simulink model "stereo_ibvs_core_before_04_kinematics_20260723_212009"  (R2025b)
settings: Solver=FixedStepDiscrete  StartTime=0.0  StopTime=inf  FixedStep=cfg.Ts  RelTol=1e-3
InitFcn:
  | cfgValid__=evalin('base','exist(''cfg'',''var'')==1 && isstruct(cfg) && all(isfield(cfg,{''Ts'',''robot'',''qInitial'',''zoomInitialSteps'',''cameraIntrinsicsStage1'',''rhoD'',''stereoBaseline'',''centerDesired'',''Kc'',''lambdaC'',''qMin'',''qMax'',''qLimitSoftMargin'',''qDotAlgorithmMax'',''stage1CalibrationReady''}))');if ~cfgValid__,modelFile__=get_param(bdroot,'FileName');modelDir__=fileparts(modelFile__);config1__=fullfile(modelDir__,'stereo_ibvs_config.m');config2__=fullfile(fileparts(modelDir__),'config','stereo_ibvs_config.m');if isfile(config1__),run(config1__);elseif isfile(config2__),run(config2__);else,error('StereoIBVS:ConfigNotFound','找不到stereo_ibvs_config.m。');end;end;clear cfgValid__ modelFile__ modelDir__ config1__ config2__
undefined symbols (not defined in the file): cfg
(part 2 of 2)

== matlab function stereo_ibvs_core_before_04_kinematics_20260723_212009/08_Zoom_Controller/08C Zoom Priority Supervisor ==
  data: scaleError input; depthErrorDelayed input; focalLengthMeasuredMm input; focalAtWorkingLowerLimit input; focalAtWorkingUpperLimit input; depthTaskWeight output; focalHeadroomMm input; focalFeasible input; validLeft input; validStereoQualified input; ekfPredictionValid input; resetSafe input; focalCommandOutwardAtWorkingLimit input; focalRateUsageGuaranteedCmd input; focalRateUsageHardCmd input; rightReacquireActive input; schedulerMode output; zoomPriorityActive output; zoomPriorityTimer output; scaleSettledTimer output; armRecoveryReason output; newDisturbanceDetected output
function [ ...
    depthTaskWeight, ...
    schedulerMode, ...
    zoomPriorityActive, ...
    zoomPriorityTimer, ...
    scaleSettledTimer, ...
    armRecoveryReason, ...
    newDisturbanceDetected] = fcn( ...
    scaleError, ...
    depthErrorDelayed, ...
    focalLengthMeasuredMm, ...
    focalAtWorkingLowerLimit, ...
    focalAtWorkingUpperLimit, ...
    focalHeadroomMm, ...
    focalFeasible, ...
    validLeft, ...
    validStereoQualified, ...
    ekfPredictionValid, ...
    resetSafe, ...
    focalCommandOutwardAtWorkingLimit, ...
    focalRateUsageGuaranteedCmd, ...
    focalRateUsageHardCmd, ...
    rightReacquireActive)
%#codegen
% V2 Zoom优先级状态机。
%
% schedulerMode:
% 0 INITIALIZE
% 1 ZOOM_FIRST
% 2 ARM_RECOVERY
% 3 FULL_TRACK
% 4 SAFE_HOLD
% 5 RIGHT_REACQUIRE

persistent mode
persistent zoomTimer
persistent settledTimer
persistent rampTimer
persistent reason
persistent disturbanceTimer
persistent validLast
persistent rateTimer

if isempty(mode)
    mode = 0;
    zoomTimer = 0;
    settledTimer = 0;
    rampTimer = 0;
    reason = 0;
    disturbanceTimer = 0;
    validLast = 0;
    rateTimer = 0;
end

if resetSafe > 0.5
    mode = 0;
    zoomTimer = 0;
    settledTimer = 0;
    rampTimer = 0;
    reason = 0;
    disturbanceTimer = 0;
    validLast = 0;
    rateTimer = 0;
end

depthTaskWeight = 0;
newDisturbanceDetected = 0;

centerValid = validLeft > 0.5;

depthReady = ...
    validStereoQualified > 0.5 && ...
    ekfPredictionValid > 0.5 && ...
    rightReacquireActive <= 0.5;

maximumScaleError = max(abs(scaleError));

if ~centerValid

    mode = 4;
    depthTaskWeight = 0;
    validLast = 0;

elseif ~depthReady

    mode = 5;
    depthTaskWeight = 0;
    validLast = 0;
    rampTimer = 0;

elseif cfg_zoomPriorityEnable <= 0.5

    mode = 3;
    depthTaskWeight = 1;

    zoomTimer = 0;
    settledTimer = 0;
    rampTimer = cfg_armDepthRampTime;

    reason = 0;
    disturbanceTimer = 0;
    validLast = 1;

else

    if validLast < 0.5 && ...
            (mode == 4 || mode == 5)

        mode = 1;

        zoomTimer = 0;
        settledTimer = 0;
        rampTimer = 0;

        reason = 0;
        disturbanceTimer = 0;
    end

    if mode == 0

        if maximumScaleError > ...
                cfg_scaleErrorEnterThreshold

            mode = 1;
            depthTaskWeight = 0;
        else
            mode = 3;
            depthTaskWeight = 1;
        end

    elseif mode == 1

        depthTaskWeight = 0;
        zoomTimer = zoomTimer + cfg_Ts;

        if maximumScaleError <= ...
                cfg_scaleErrorExitThreshold

            settledTimer = settledTimer + cfg_Ts;
        else
            settledTimer = 0;
        end

        if any(focalRateUsageGuaranteedCmd >= 1)
            rateTimer = rateTimer + cfg_Ts;
        else
            rateTimer = 0;
        end

        if any(focalRateUsageHardCmd >= 1)

            mode = 2;
            reason = 6;
            rampTimer = 0;

        elseif rateTimer >= ...
                cfg_disturbanceConfirmTime && ...
                maximumScaleError > ...
                cfg_scaleErrorExitThreshold

            mode = 2;
            reason = 5;
            rampTimer = 0;

        elseif settledTimer >= ...
                cfg_scaleSettledHoldTime

            mode = 2;
            reason = 1;
            rampTimer = 0;

        elseif any( ...
                focalCommandOutwardAtWorkingLimit > 0.5)

            mode = 2;
            reason = 7;
            rampTimer = 0;

        elseif zoomTimer >= ...
                cfg_disturbanceConfirmTime && ...
                any(focalFeasible < 0.5)

            mode = 2;
            reason = 3;
            rampTimer = 0;

        elseif zoomTimer >= cfg_zoomOnlyMaxTime

            mode = 2;
            reason = 4;
            rampTimer = 0;
        end

    elseif mode == 2

        rampTimer = min( ...
            rampTimer + cfg_Ts, ...
            cfg_armDepthRampTime);

        rampFraction = min(max( ...
            rampTimer / max( ...
                cfg_armDepthRampTime, ...
                cfg_Ts), ...
            0), 1);

        depthTaskWeight = ...
            rampFraction * rampFraction * ...
            (3 - 2*rampFraction);

        if depthTaskWeight >= 1 - 1e-6
            mode = 3;
            depthTaskWeight = 1;
            disturbanceTimer = 0;
        end

    elseif mode == 3

        depthTaskWeight = 1;

        if maximumScaleError >= ...
                cfg_scaleErrorEnterThreshold

            depthTaskWeight = 0;
            disturbanceTimer = ...
                disturbanceTimer + cfg_Ts;
        else
            disturbanceTimer = 0;
        end

        if disturbanceTimer >= ...
                cfg_disturbanceConfirmTime

            mode = 1;
            depthTaskWeight = 0;

            zoomTimer = 0;
            settledTimer = 0;
            rampTimer = 0;

            reason = 0;
            disturbanceTimer = 0;

            newDisturbanceDetected = 1;
        end

    else

        mode = 1;
        depthTaskWeight = 0;

        zoomTimer = 0;
        settledTimer = 0;
        rampTimer = 0;

        reason = 0;
    end

    validLast = 1;
end

schedulerMode = mode;
zoomPriorityActive = double(mode == 1);

zoomPriorityTimer = zoomTimer;
scaleSettledTimer = settledTimer;
armRecoveryReason = reason;

%% 数值保护
if any(~isfinite([
        depthTaskWeight
        schedulerMode
        zoomPriorityTimer
        scaleSettledTimer
        depthErrorDelayed
        focalLengthMeasuredMm
        focalHeadroomMm
        focalAtWorkingLowerLimit
        focalAtWorkingUpperLimit]))

    depthTaskWeight = 0;
    schedulerMode = 4;
    zoomPriorityActive = 0;
    newDisturbanceDetected = 0;
end
end

== matlab function stereo_ibvs_core_before_04_kinematics_20260723_212009/04_FR3_Camera_Kinematics/Express Jacobian in Left Camera ==
  data: q input; pWCL output; cfg_T_W_B input; cfg_fr3OriginXYZ input; cfg_fr3OriginRPY input; cfg_fr3Axis input; cfg_fr3Joint8OriginXYZ input; cfg_fr3Joint8OriginRPY input; cfg_T_link8_CL input; cfg_T_CL_CR input; cfg_numericalEpsilon input; RWCL output; pWCR output; RWCR output; JL output; JR output; kinematicsValid output
function [ ...
    pWCL, ...
    RWCL, ...
    pWCR, ...
    RWCR, ...
    JL, ...
    JR, ...
    kinematicsValid] = fcn(q, cfg_T_W_B, cfg_fr3OriginXYZ, cfg_fr3OriginRPY, cfg_fr3Axis, cfg_fr3Joint8OriginXYZ, cfg_fr3Joint8OriginRPY, cfg_T_link8_CL, cfg_T_CL_CR, cfg_numericalEpsilon)
%#codegen
% V2 FR3双目相机运动学。
%
% 输入：
% q：FR3七关节角，7×1，单位rad。
%
% 输出：
% pWCL、RWCL：左相机在世界坐标系中的位置和姿态。
% pWCR、RWCR：右相机在世界坐标系中的位置和姿态。
% JL、JR：左右相机坐标系表达的相机Jacobian，
%          排列顺序为[线速度; 角速度]。
% kinematicsValid：运动学结果是否有效。

%% 固定尺寸输出初始化
pWCL = zeros(3,1);
RWCL = eye(3);

pWCR = zeros(3,1);
RWCR = eye(3);

JL = zeros(6,7);
JR = zeros(6,7);

kinematicsValid = false;

%% 输入检查
if any(~isfinite(q))
    return;
end

%% FR3正运动学
T = cfg_T_W_B;

jointOriginsW = zeros(3,7);
jointAxesW = zeros(3,7);

for jointIndex = 1:7

    % 当前关节固定原点变换
    T = T * makeTransform( ...
        cfg_fr3OriginXYZ(:,jointIndex), ...
        cfg_fr3OriginRPY(:,jointIndex));

    jointOriginsW(:,jointIndex) = T(1:3,4);

    axisLocal = cfg_fr3Axis(:,jointIndex);
    axisNorm = norm(axisLocal);

    if ~isfinite(axisNorm) || ...
            axisNorm <= cfg_numericalEpsilon
        return;
    end

    jointAxesW(:,jointIndex) = ...
        T(1:3,1:3) * axisLocal;

    % 当前关节转动
    T = T * axisRotation(axisLocal,q(jointIndex));
end

%% link8固定变换
T_W_link8 = T * makeTransform( ...
    cfg_fr3Joint8OriginXYZ, ...
    cfg_fr3Joint8OriginRPY);

%% 左右相机位姿
T_W_CL = T_W_link8 * cfg_T_link8_CL;
T_W_CR = T_W_CL * cfg_T_CL_CR;

pWCL = T_W_CL(1:3,4);
RWCL = T_W_CL(1:3,1:3);

pWCR = T_W_CR(1:3,4);
RWCR = T_W_CR(1:3,1:3);

%% 左相机光心世界坐标Jacobian
JWLeft = zeros(6,7);

for jointIndex = 1:7

    JWLeft(1:3,jointIndex) = cross( ...
        jointAxesW(:,jointIndex), ...
        pWCL-jointOriginsW(:,jointIndex));

    JWLeft(4:6,jointIndex) = ...
        jointAxesW(:,jointIndex);
end

%% 转换到左相机坐标系
R_CL_W = RWCL';

JL = [
    R_CL_W, zeros(3,3)
    zeros(3,3), R_CL_W
    ] * JWLeft;

%% 从左相机Jacobian转换为右相机Jacobian
R_CL_CR = cfg_T_CL_CR(1:3,1:3);
p_CL_CR = cfg_T_CL_CR(1:3,4);

JR = [
    R_CL_CR', -R_CL_CR' * skew3(p_CL_CR)
    zeros(3,3), R_CL_CR'
    ] * JL;

%% 有限值和旋转矩阵检查
if any(~isfinite(pWCL)) || ...
        any(~isfinite(RWCL(:))) || ...
        any(~isfinite(pWCR)) || ...
        any(~isfinite(RWCR(:))) || ...
        any(~isfinite(JL(:))) || ...
        any(~isfinite(JR(:)))

    pWCL = zeros(3,1);
    RWCL = eye(3);
    pWCR = zeros(3,1);
    RWCR = eye(3);
    JL = zeros(6,7);
    JR = zeros(6,7);
    return;
end

rotationTolerance = max( ...
    1e-6, ...
    100*cfg_numericalEpsilon);

if norm(RWCL'*RWCL-eye(3),'fro') > rotationTolerance || ...
        norm(RWCR'*RWCR-eye(3),'fro') > rotationTolerance || ...
        abs(det(RWCL)-1) > rotationTolerance || ...
        abs(det(RWCR)-1) > rotationTolerance
    return;
end

kinematicsValid = true;

end


function T = makeTransform(xyz,rpy)

T = eye(4);

T(1:3,1:3) = ...
    rotz3(rpy(3)) * ...
    roty3(rpy(2)) * ...
    rotx3(rpy(1));

T(1:3,4) = xyz;

end


function T = axisRotation(axis,q)

axisNorm = norm(axis);
unitAxis = axis / axisNorm;

K = skew3(unitAxis);

R = eye(3) + ...
    sin(q)*K + ...
    (1-cos(q))*(K*K);

T = eye(4);
T(1:3,1:3) = R;

end


function R = rotx3(angle)

c = cos(angle);
s = sin(angle);

R = [
    1, 0, 0
    0, c, -s
    0, s, c
    ];

end


function R = roty3(angle)

c = cos(angle);
s = sin(angle);

R = [
    c, 0, s
    0, 1, 0
    -s, 0, c
    ];

end


function R = rotz3(angle)

c = cos(angle);
s = sin(angle);

R = [
    c, -s, 0
    s, c, 0
    0, 0, 1
    ];

end


function S = skew3(vector)

S = [
    0, -vector(3), vector(2)
    vector(3), 0, -vector(1)
    -vector(2), vector(1), 0
    ];

end

== matlab function stereo_ibvs_core_before_04_kinematics_20260723_212009/03_Feature_Processing/Normalize and Validate Features ==
  data: normalizedFeatureMeasured output size=[4 1]; pixelMeasurement input size=[4 1]; cLMeasured output size=[2 1]; scaleMeasuredRaw input size=[2 1]; cRMeasured output size=[2 1]; scaleMeasured output size=[2 1]; zMeasured output size=[3 1]; fxMeasuredPx input size=[2 1]; fyMeasuredPx input size=[2 1]; validLeft input size=[1 1]; validRight input size=[1 1]; visionMeasurementNew input size=[1 1]; resetSafe input size=[1 1]; xLeftMeasured output size=[1 1]; yLeftMeasured output size=[1 1]; xRightMeasured output size=[1 1]; disparityNormalized output size=[1 1]; rhoMeasured output size=[1 1]; validDisparity output size=[1 1]; stereoMeasurementEnable output size=[1 1]; validStereoQualified output size=[1 1]; rightReacquireActive output size=[1 1]; rightReacquireCount output size=[1 1]; uRightMeasured output size=[1 1]
function [ ...
    normalizedFeatureMeasured, ...
    cLMeasured, ...
    cRMeasured, ...
    scaleMeasured, ...
    zMeasured, ...
    xLeftMeasured, ...
    yLeftMeasured, ...
    xRightMeasured, ...
    disparityNormalized, ...
    rhoMeasured, ...
    validDisparity, ...
    stereoMeasurementEnable, ...
    validStereoQualified, ...
    rightReacquireActive, ...
    rightReacquireCount, ...
    uRightMeasured] = fcn( ...
    pixelMeasurement, ...
    scaleMeasuredRaw, ...
    fxMeasuredPx, ...
    fyMeasuredPx, ...
    validLeft, ...
    validRight, ...
    visionMeasurementNew, ...
    resetSafe)
%#codegen
% V2实机视觉测量提取与双目有效性管理。
%
% pixelMeasurement:
% [uL; vL; uR; vR]
%
% scaleMeasuredRaw:
% [scaleL; scaleR]
%
% fxMeasuredPx:
% [fxL; fxR]
%
% fyMeasuredPx:
% [fyL; fyR]
%
% zMeasured:
% [xLeftMeasured; yLeftMeasured; rhoMeasured]

%% 固定尺寸输出
normalizedFeatureMeasured = zeros(4,1);

cLMeasured = zeros(2,1);
cRMeasured = zeros(2,1);
scaleMeasured = zeros(2,1);

zMeasured = zeros(3,1);

xLeftMeasured = 0;
yLeftMeasured = 0;
xRightMeasured = 0;

disparityNormalized = 0;
rhoMeasured = 0;

validDisparity = 0;
stereoMeasurementEnable = 0;
validStereoQualified = 0;

rightReacquireActive = 0;
rightReacquireCount = 0;

uRightMeasured = 0;

%% 右相机重捕获状态
persistent consecutiveValid reacquire

if isempty(consecutiveValid)
    consecutiveValid = 0;
    reacquire = 1;
end

%% 输入整理
pixels = reshape(pixelMeasurement,4,1);
scales = reshape(scaleMeasuredRaw,2,1);
fx = reshape(fxMeasuredPx,2,1);
fy = reshape(fyMeasuredPx,2,1);

inputFinite = ...
    all(isfinite(pixels)) && ...
    all(isfinite(scales)) && ...
    all(isfinite(fx)) && ...
    all(isfinite(fy));

if inputFinite
    uL = pixels(1);
    vL = pixels(2);
    uR = pixels(3);
    vR = pixels(4);

    uRightMeasured = uR;

    leftIntrinsicsValid = ...
        fx(1) > cfg_numericalEpsilon && ...
        fy(1) > cfg_numericalEpsilon;

    rightIntrinsicsValid = ...
        fx(2) > cfg_numericalEpsilon && ...
        fy(2) > cfg_numericalEpsilon;

    leftFeatureValid = ...
        validLeft > 0.5 && ...
        leftIntrinsicsValid;

    rightFeatureValid = ...
        validRight > 0.5 && ...
        rightIntrinsicsValid;

    %% 像素坐标归一化
    if leftIntrinsicsValid
        cLMeasured = [
            (uL - cfg_cxL) / fx(1)
            (vL - cfg_cyL) / fy(1)
        ];
    end

    if rightIntrinsicsValid
        cRMeasured = [
            (uR - cfg_cxR) / fx(2)
            (vR - cfg_cyR) / fy(2)
        ];
    end

    if leftFeatureValid && scales(1) > 0
        scaleMeasured(1) = scales(1);
    end

    if rightFeatureValid && scales(2) > 0
        scaleMeasured(2) = scales(2);
    end

    normalizedFeatureMeasured = [
        cLMeasured
        cRMeasured
    ];

    xLeftMeasured = cLMeasured(1);
    yLeftMeasured = cLMeasured(2);
    xRightMeasured = cRMeasured(1);

    %% 双目视差与逆深度测量
    disparityNormalized = ...
        xLeftMeasured - xRightMeasured;

    candidateRho = 0;

    if cfg_baseline > cfg_numericalEpsilon
        candidateRho = ...
            disparityNormalized / cfg_baseline;
    end

    validDisparity = double( ...
        leftFeatureValid && ...
        rightFeatureValid && ...
        isfinite(candidateRho) && ...
        disparityNormalized > cfg_disparityMin && ...
        candidateRho >= cfg_rhoMin && ...
        candidateRho <= cfg_rhoMax);

    if validDisparity > 0.5
        rhoMeasured = candidateRho;
    end

    zMeasured = [
        xLeftMeasured
        yLeftMeasured
        rhoMeasured
    ];
end

%% 最终有限值保护
if any(~isfinite(normalizedFeatureMeasured))
    normalizedFeatureMeasured = zeros(4,1);
    cLMeasured = zeros(2,1);
    cRMeasured = zeros(2,1);

    zMeasured = zeros(3,1);

    xLeftMeasured = 0;
    yLeftMeasured = 0;
    xRightMeasured = 0;

    disparityNormalized = 0;
    rhoMeasured = 0;
    validDisparity = 0;
end

%% 双目资格与右相机重捕获管理
rawStereoValid = ...
    inputFinite && ...
    validLeft > 0.5 && ...
    validRight > 0.5 && ...
    validDisparity > 0.5;

if resetSafe > 0.5
    consecutiveValid = 0;
    reacquire = 1;

elseif visionMeasurementNew > 0.5
    if rawStereoValid
        consecutiveValid = min( ...
            consecutiveValid + 1, ...
            cfg_rightReacquireValidSamples);
    else
        consecutiveValid = 0;
    end

    if ~rawStereoValid
        reacquire = 1;
    elseif consecutiveValid >= ...
            cfg_rightReacquireValidSamples
        reacquire = 0;
    end
end

validStereoQualified = double( ...
    rawStereoValid && ...
    consecutiveValid >= ...
        cfg_rightReacquireValidSamples);

% 只允许每个新视觉测量触发一次EKF校正。
stereoMeasurementEnable = double( ...
    visionMeasurementNew > 0.5 && ...
    validStereoQualified > 0.5 && ...
    resetSafe <= 0.5);

rightReacquireActive = double( ...
    validLeft > 0.5 && ...
    reacquire > 0.5);

rightReacquireCount = consecutiveValid;
end

== matlab function stereo_ibvs_core_before_04_kinematics_20260723_212009/02_Camera_Model/Zoom Position to Camera Intrinsics ==
  data: zoomPositionSteps input; cameraIntrinsics output; intrinsicsFixed input; focalLengthPx output; cameraModelValid output
function [cameraIntrinsics,focalLengthPx,cameraModelValid] = ...
    fcn(zoomPositionSteps,intrinsicsFixed)
%#codegen
% 代码作用：
% Stage 1暂时不根据步进电机位置改变相机内参。
% 本函数检查输入是否合法，并输出左右相机的固定内参。
% Stage 5加入变焦后，再将这里替换为“电机步数到相机内参”的标定模型。

% 输入参数含义：
% zoomPositionSteps：
% 左右变焦步进电机的累计位置，格式为：
% [leftSteps; rightSteps]
%
% intrinsicsFixed：
% Stage 1使用的固定相机内参，格式为：
% [fxL; fyL; cxL; cyL; fxR; fyR; cxR; cyR]

% 输出参数含义：
% cameraIntrinsics：
% 左右相机当前使用的内参，格式为：
% [fxL; fyL; cxL; cyL; fxR; fyR; cxR; cyR]
%
% focalLengthPx：
% 左右相机水平方向焦距，单位为像素，格式为：
% [fxL; fxR]
%
% cameraModelValid：
% 相机模型是否有效。有效为1，无效为0。

cameraIntrinsics = zeros(8,1);
focalLengthPx = zeros(2,1);
cameraModelValid = 0;

steps = reshape(zoomPositionSteps,2,1);
intrinsics = reshape(intrinsicsFixed,8,1);

% 检查输入中是否存在NaN或Inf。
if any(~isfinite(steps)) || any(~isfinite(intrinsics))
    return;
end

fxL = intrinsics(1);
fyL = intrinsics(2);
fxR = intrinsics(5);
fyR = intrinsics(6);

% 焦距必须为正数。
if fxL <= 0 || fyL <= 0 || fxR <= 0 || fyR <= 0
    return;
end

% Stage 1直接采用固定内参。
cameraIntrinsics = intrinsics;
focalLengthPx = [fxL; fxR];
cameraModelValid = 1;
end

== matlab function stereo_ibvs_core_before_04_kinematics_20260723_212009/07_Arm_Priority_Controller/Final Arm Priority Controller ==
  data: q input double size=[7 1]; qDotCmd output double size=[7 1]; cLMeasured input double size=[2 1]; rhoHatL input double size=[1 1]; vHatLeft input double size=[3 1]; JL input double size=[6 7]; cLd input double size=[2 1]; rhoD input double size=[1 1]; validLeft input double size=[1 1]; ekfPredictionValid input double size=[1 1]; centerEnable input double size=[1 1]; depthEnable input double size=[1 1]; armEnable input double size=[1 1]; depthTaskWeight input double size=[1 1]; cfg_numericalEpsilon input double size=[1 1]; cfg_robustEnable input double size=[1 1]; cfg_betaC input double size=[1 1]; cfg_epsilonC input double size=[1 1]; cfg_Kc input double size=[2 2]; cfg_lambdaC input double size=[1 1]; cfg_betaRho input double size=[1 1]; cfg_epsilonRho input double size=[1 1]; cfg_kRho input double size=[1 1]; cfg_lambdaRho input double size=[1 1]; cfg_nullspaceEnable input double size=[1 1]; cfg_kNull input double size=[1 1]; cfg_qMid input double size=[7 1]; cfg_leftOnlyCenterControlEnable input double size=[1 1]; centerError output double size=[2 1]; depthError output double size=[1 1]; rcondJc output double size=[1 1]; rcondArho output double size=[1 1]; qDotCenter output double size=[7 1]; qDotDepthRaw output double size=[7 1]; qDotDepthWeighted output double size=[7 1]; qDotNullUsed output double size=[7 1]
function [qDotCmd,centerError,depthError,rcondJc,rcondArho,qDotCenter,qDotDepthRaw,qDotDepthWeighted,qDotNullUsed] = ...
    fcn(q,cLMeasured,rhoHatL,vHatLeft,JL,cLd,rhoD,validLeft,ekfPredictionValid,centerEnable,depthEnable,armEnable,depthTaskWeight, ...
    cfg_numericalEpsilon,cfg_robustEnable,cfg_betaC,cfg_epsilonC,cfg_Kc,cfg_lambdaC,cfg_betaRho,cfg_epsilonRho,cfg_kRho,cfg_lambdaRho,cfg_nullspaceEnable,cfg_kNull,cfg_qMid,cfg_leftOnlyCenterControlEnable)
%#codegen
% 代码作用：
% 左相机归一化中心为主任务，逆深度为次任务。
% 支持目标速度前馈、鲁棒项、阻尼伪逆和关节中位零空间任务。

qDotCmd = zeros(7,1);
centerError = zeros(2,1);
depthError = 0;
rcondJc = 0;
rcondArho = 0;
qDotCenter = zeros(7,1);
qDotDepthRaw = zeros(7,1);
qDotDepthWeighted = zeros(7,1);
qDotNullUsed = zeros(7,1);

x = cLMeasured(1);
y = cLMeasured(2);
rho = rhoD;
vFeed = zeros(3,1);

if ekfPredictionValid > 0.5 && ...
        isfinite(rhoHatL) && rhoHatL > 0 && ...
        all(isfinite(vHatLeft))
    rho = max(rhoHatL,cfg_numericalEpsilon);
    vFeed = vHatLeft;
end

centerError = [x;y] - cLd;
depthError = rho - rhoD;

Lc = [
    -rho, 0, x*rho, x*y, -(1+x*x), y
    0, -rho, y*rho, 1+y*y, -x*y, -x
];

Hc = rho*[1 0 -x;0 1 -y];
bhatC = Hc*vFeed;
Jc = Lc*JL;

rc = zeros(2,1);
if cfg_robustEnable > 0.5
    rc = cfg_betaC*centerError / ...
        (sqrt(centerError'*centerError)+cfg_epsilonC);
end

nuC = -cfg_Kc*centerError - bhatC - rc;
Gc = Jc*Jc' + cfg_lambdaC^2*eye(2);
JcSharp = Jc'/Gc;
qC = JcSharp*nuC;
Nc = eye(7)-JcSharp*Jc;
rcondJc = det(Gc) / ...
    (trace(Gc)*trace(Gc)+cfg_numericalEpsilon);
qDotCenter = qC;

Lrho = [0 0 rho*rho rho*y -rho*x 0];
Hrho = [0 0 -rho*rho];
Jrho = Lrho*JL;
bhatRho = Hrho*vFeed;

rr = 0;
if cfg_robustEnable > 0.5
    rr = cfg_betaRho*depthError / ...
        (abs(depthError)+cfg_epsilonRho);
end

nuRho = -cfg_kRho*depthError-bhatRho-rr;
A = Jrho*Nc;
denom = A*A'+cfg_lambdaRho^2;
rcondArho = denom/(1+denom);

w = min(max(depthTaskWeight,0),1) * ...
    double(ekfPredictionValid > 0.5);
qDotDepthRaw = Nc*A'*((nuRho-Jrho*qC)/denom);
qDotDepthWeighted = w*qDotDepthRaw;

qDot0 = zeros(7,1);
if cfg_nullspaceEnable > 0.5
    qDot0 = -cfg_kNull*(q-cfg_qMid);
end

ArhoDagger = A'/denom;
NcRho = Nc*(eye(7)-ArhoDagger*A);
Nnull = (1-w)*Nc+w*NcRho;
qDotNullUsed = Nnull*qDot0;

if centerEnable > 0.5
    qDotCmd = qDotCenter+qDotNullUsed;
end

if centerEnable > 0.5 && depthEnable > 0.5
    qDotCmd = qDotCenter+qDotDepthWeighted+qDotNullUsed;
end

if centerEnable <= 0.5 && depthEnable > 0.5
    d = Jrho*Jrho'+cfg_lambdaRho^2;
    qDotDepthRaw = Jrho'*(nuRho/d);
    qDotDepthWeighted = w*qDotDepthRaw;
    qDotCenter = zeros(7,1);
    qDotNullUsed = zeros(7,1);
    qDotCmd = qDotDepthWeighted;
end

centerAllowed = validLeft > 0.5 && ...
    cfg_leftOnlyCenterControlEnable > 0.5;

if ~centerAllowed || armEnable <= 0.5
    qDotCmd = zeros(7,1);
    qDotCenter = zeros(7,1);
    qDotDepthWeighted = zeros(7,1);
    qDotNullUsed = zeros(7,1);
end

if any(~isfinite(qDotCmd))
    qDotCmd = zeros(7,1);
end
end
